simulink model "Dynamic_RR_2019b"  (Simulink 10.0)
settings: Solver=VariableStepAuto  StartTime=0.0  StopTime=1000  FixedStep=1e-2  RelTol=1e-3
undefined symbols (not defined in the file or in its folder): a_11, a_12, b_11, b_12, pi_param, pi_param_hat_0, q0_1, q0_2, qInitial_0, wf
libraries: dspfactors x1
settings Model: Creator=Stefano  LastModifiedBy=dnann
settings DataIOCC: SaveFormat=Dataset  ReturnWorkspaceOutputs=on
settings OptimizationCC: LifeSpan=auto
settings DebuggingCC: UnderspecifiedInitializationDetection=Simplified  MergeDetectMultiDrivingBlocksExec=error  SFUnexpectedBacktrackingDiag=error  SFNoUnconditionalDefaultTransitionDiag=error  SFExecutionAtInitializationDiag=warning  ArithmeticOperatorsInVariantConditions=error
settings HardwareCC: ProdBitPerPointer=64  ProdBitPerSizeT=64  ProdBitPerPtrDiffT=64  ProdLargestAtomicFloat=Float  ProdIntDivRoundTo=Zero  ProdEndianess=LittleEndian  ProdWordSize=64  ProdHWDeviceType=Intel->x86-64 (Windows64)
settings ModelReferenceCC: PropagateSignalLabelsOutOfModel=on
settings SFSimCC: SimUseLocalCustomCode=on  CustomCodeUndefinedFunction=FilterOut
settings RTWCC: RTWUseLocalCustomCode=on
settings CodeAppCC: StateflowObjectComments=off
settings GRTTargetCC: TargetLangStandard=C99 (ISO)  CombineOutputUpdateFcns=on  GRTInterface=off
settings ConfigComp: CovMetricSettings=dwe  CovHtmlReporting=off  CovSaveCumulativeToWorkspaceVar=off  CovSaveSingleToWorkspaceVar=off

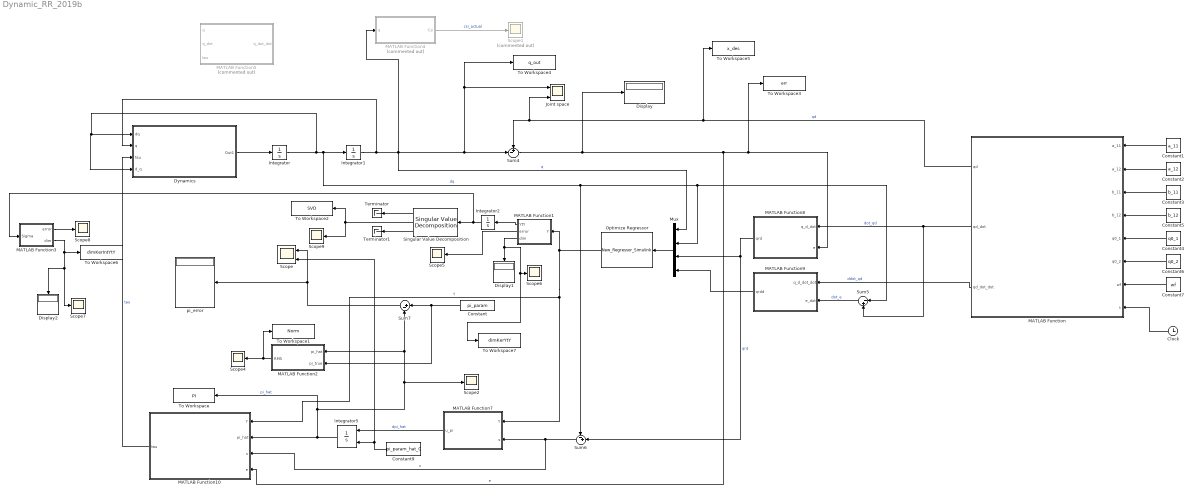
== system Dynamic_RR_2019b ==
  Clock : Clock
  Constant : Constant  Value=pi_param
  Constant1 : Constant  Value=a_11
  Constant2 : Constant  Value=a_12
  Constant3 : Constant  Value=b_11
  Constant4 : Constant  Value=q0_1
  Constant5 : Constant  Value=b_12
  Constant6 : Constant  Value=q0_2
  Constant7 : Constant  Value=wf
  Constant9 : Constant  Value=pi_param_hat_0
  Display : Display
  Display1 : Display
  Display2 : Display
  Dynamics : Subsystem
  Integrator : Integrator  InitialCondition=qInitial_0
  Integrator1 : Integrator  InitialCondition=[0,0]'
  Integrator2 : Integrator
  Integrator5 : Integrator  InitialConditionSource=external
  Joint space : Scope  NumInputPorts=2
  MATLAB Function : MATLAB Function  TreatAsAtomicUnit=on
  MATLAB Function1 : MATLAB Function  TreatAsAtomicUnit=on
  MATLAB Function10 : MATLAB Function  TreatAsAtomicUnit=on
  MATLAB Function2 : MATLAB Function  TreatAsAtomicUnit=on
  MATLAB Function3 : MATLAB Function  TreatAsAtomicUnit=on
  MATLAB Function4 : MATLAB Function  Commented=on  TreatAsAtomicUnit=on
  MATLAB Function5 : MATLAB Function  Commented=on  TreatAsAtomicUnit=on
  MATLAB Function7 : MATLAB Function  TreatAsAtomicUnit=on
  MATLAB Function8 : MATLAB Function  TreatAsAtomicUnit=on
  MATLAB Function9 : MATLAB Function  TreatAsAtomicUnit=on
  Mux : Mux
  "Optimize Regressor " : MATLABFcn  MATLABFcn=New_Regressor_Simulink  OutputDimensions=[2,6]  Output1D=off
  Scope : Scope  NumInputPorts=2
  Scope1 : Scope  Commented=on
  Scope{2,4..9} (7 alike) : Scope
  Singular Value Decomposition : dspfactors/Singular Value Decomposition  wantv=on  wanterr=off  SimulateUsing=Interpreted execution
      settings: SourceProductBaseCode=DS
  Sum4 : Sum  Inputs=+-|
  Sum5 : Sum  Inputs=|-+
  Sum6 : Sum  Inputs=-+|
  Sum7 : Sum  Inputs=|+-
  Terminator : Terminator
  Terminator1 : Terminator
  To Workspace : ToWorkspace  VariableName=PI  SaveFormat=Timeseries  SampleTime=-1
  To Workspace1 : ToWorkspace  VariableName=Norm  SaveFormat=Timeseries  SampleTime=-1
  To Workspace2 : ToWorkspace  VariableName=SVD  SaveFormat=Timeseries  SampleTime=-1
  To Workspace3 : ToWorkspace  VariableName=err  SaveFormat=Timeseries  SampleTime=-1
  To Workspace4 : ToWorkspace  VariableName=q_out  SaveFormat=Timeseries  SampleTime=-1
  To Workspace5 : ToWorkspace  VariableName=x_des  SaveFormat=Timeseries  SampleTime=-1
  To Workspace6 : ToWorkspace  VariableName=dimKerIntYtY  SaveFormat=Timeseries  SampleTime=-1
  To Workspace7 : ToWorkspace  VariableName=dimKerYtY  SaveFormat=Timeseries  SampleTime=-1
  pi_error : Display
  wires:
  Sum6/1 -> MATLAB Function10/3(s), MATLAB Function7/2(s)  "s"
  Sum4/1 -> Display/1, To Workspace3/1, MATLAB Function8/2(e), MATLAB Function10/4(e)  "e"
  Sum5/1 -> MATLAB Function9/2(e_dot)  "dot_e"
  MATLAB Function7/1(u_pi) -> Integrator5/1  "dpi_hat"
  Integrator5/1 -> MATLAB Function10/2(pi_hat), To Workspace/1, Scope2/1, Sum7/2, MATLAB Function2/1(pi_hat)  "pi_hat"
  Integrator/1 -> Sum5/1, Mux/2, Sum6/1, Integrator1/1, Dynamics/1(dq), Dynamics/4(d_q)  "dq"
  Constant9/1 -> Scope/2, Integrator5/2
  MATLAB Function8/1(qrd) -> Sum6/2, Mux/3  "qrd"
  Mux/1 -> "Optimize Regressor "/1
  MATLAB Function9/1(qrdd) -> Mux/4
  Constant/1 -> MATLAB Function2/2(pi_true), Sum7/1
  Sum7/1 -> pi_error/1, Scope/1
  Integrator1/1 -> Dynamics/2(q), Joint space/1, To Workspace4/1, Sum4/2, MATLAB Function4/1(q), Mux/1  "q"
  "Optimize Regressor "/1 -> MATLAB Function10/1(Y), MATLAB Function7/1(Y), MATLAB Function1/1(Y)  "Y"
  MATLAB Function/1(qd) -> To Workspace5/1, Joint space/2, Sum4/1  "qd"
  MATLAB Function/2(qd_dot) -> Sum5/2, MATLAB Function8/1(q_d_dot)  "dot_qd"
  MATLAB Function/3(qd_dot_dot) -> MATLAB Function9/1(q_d_dot_dot)  "ddot_qd"
  MATLAB Function4/1(Csi) -> Scope1/1  "csi_actual"
  Constant1/1 -> MATLAB Function/1(a_11)
  Constant2/1 -> MATLAB Function/2(a_12)
  Constant3/1 -> MATLAB Function/3(b_11)
  Constant5/1 -> MATLAB Function/4(b_12)
  Constant4/1 -> MATLAB Function/5(q0_1)
  Constant6/1 -> MATLAB Function/6(q0_2)
  Constant7/1 -> MATLAB Function/7(wf)
  Clock/1 -> MATLAB Function/8(t)
  MATLAB Function1/1(YtY) -> Integrator2/1
  Singular Value Decomposition/2 -> Scope9/1, To Workspace2/1
  Singular Value Decomposition/1 -> Terminator/1
  Singular Value Decomposition/3 -> Terminator1/1
  Integrator2/1 -> MATLAB Function3/1(Sigma), Singular Value Decomposition/1
  MATLAB Function2/1(RMS) -> To Workspace1/1, Scope4/1
  MATLAB Function10/1(tau) -> Dynamics/3(tau)  "tau"
  Dynamics/1(Out1) -> Integrator/1
  MATLAB Function1/2(error) -> Scope5/1
  MATLAB Function1/3(dim) -> To Workspace7/1, Scope6/1, Display1/1
  MATLAB Function3/2(dim) -> Display2/1, Scope7/1, To Workspace6/1
  MATLAB Function3/1(error) -> Scope8/1

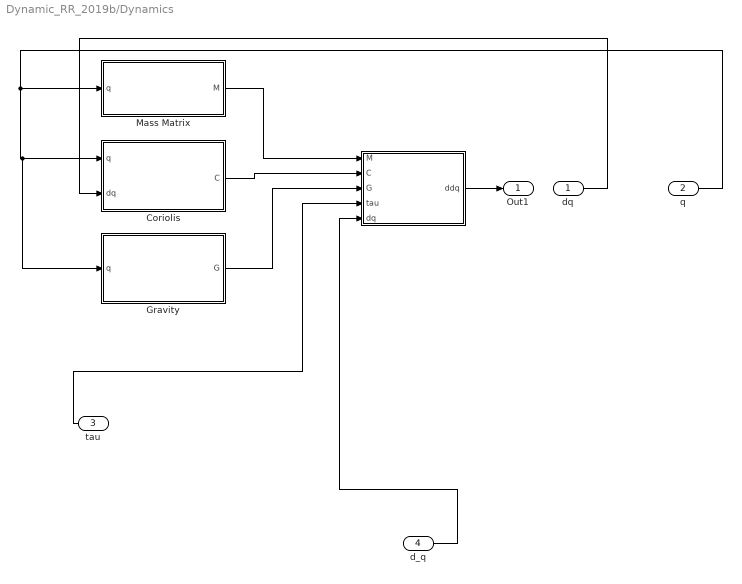
== system Dynamic_RR_2019b/Dynamics ==
  dq : Inport
  q : Inport  Port=2
  tau : Inport  Port=3
  d_q : Inport  Port=4
  " " : MATLAB Function  TreatAsAtomicUnit=on
  "Coriolis " : MATLAB Function  TreatAsAtomicUnit=on
  "Gravity " : MATLAB Function  TreatAsAtomicUnit=on
  "Mass Matrix " : MATLAB Function  TreatAsAtomicUnit=on
  Out1 : Outport
  wires:
  q/1 -> "Gravity "/1(q), "Coriolis "/1(q), "Mass Matrix "/1(q)
  tau/1 -> " "/4(tau)
  "Coriolis "/1(C) -> " "/2(C)
  "Mass Matrix "/1(M) -> " "/1(M)
  "Gravity "/1(G) -> " "/3(G)
  " "/1(ddq) -> Out1/1
  dq/1 -> "Coriolis "/2(dq)
  d_q/1 -> " "/5(dq)

== matlab function MATLAB Function1 ==
  data: Y input double; YtY output double; error output double; dim output double
function [YtY, error,dim] = fcn(Y)

YtY = Y.'*Y;

error = 0;
ker = null(YtY);
dim = 0;

if ker~=0 
    error = 1;
    dim = rank(ker);
end

== matlab function MATLAB Function ==
  data: a_11 input double; qd output double; a_12 input double; b_11 input double; b_12 input double; q0_1 input double; q0_2 input double; wf input double; t input double; qd_dot output double; qd_dot_dot output double
function [qd,qd_dot,qd_dot_dot] = De_Luca_Fourier(a_11,a_12,b_11,b_12,q0_1,q0_2,wf,t)


qd1 = q0_1 - (b_11*cos(t*wf))/wf + (a_11*sin(t*wf))/wf;
qd2 = q0_2 - (b_12*cos(t*wf))/wf + (a_12*sin(t*wf))/wf;

qd = [qd1;qd2];


qd_dot1 = a_11*cos(t*wf) + b_11*sin(t*wf);
qd_dot2 = a_12*cos(t*wf) + b_12*sin(t*wf);

qd_dot = [qd_dot1; qd_dot2];

qd_dot_dot1 = b_11*wf*cos(t*wf) - a_11*wf*sin(t*wf);
qd_dot_dot2 = b_12*wf*cos(t*wf) - a_12*wf*sin(t*wf);

qd_dot_dot = [qd_dot_dot1; qd_dot_dot2];

== matlab function MATLAB Function2 ==
  data: pi_hat input double; RMS output double; pi_true input double
function RMS = Norm(pi_hat,pi_true)

RMS = norm(pi_true - pi_hat);

== matlab function Dynamics/Mass Matrix  ==
  data: q input double; M output double
function M = RR_mass_matrix(q)

% Basic params
g = 9.81;

% Manipulator params
m1 = 1;
m2 = 1;

a1=1;
a2=1;

l1=a1/2;
l2=a2/2;

Izz1 = (1/12)*m1*a1^2;
Izz2 = (1/12)*m2*a2^2;

% Basic expressions for dynamics
Alpha = Izz1 + Izz2 + m1*(l1)^2 + m2*(a1^2+l2^2);
Beta = m2*a1*l2;
Delta = Izz2 +m2*l2^2;

% Mass matrix
M = [Alpha + 2* Beta *cos(q(2)), Delta + Beta *cos(q(2));
     Delta + Beta *cos(q(2)),    Delta];

end

== matlab function MATLAB Function5 ==
  data: q input double; q_dot_dot output double; q_dot input double; tau input double
function q_dot_dot = Forward_Dynamics(q,q_dot,tau)

q1 = q(1);
q2 = q(2);
dq1 = q_dot(1);
dq2 = q_dot(2);
%Properties of the manipulator

m1 = 1;%links mass
m2 = 1;

g = 9.81; %gravity

%COM

l1=0.5;
l2=0.5;

%lenght of the links

a1 = 1;
a2 = 1;

%Inertia respect to the center of mass 

Izz1 = (1/12)*m1*l1^2;
Izz2 = (1/12)*m2*l2^2;

%Inertia Matrix 

b11 = Izz1 + Izz2 + m1*l1^2 + m2*(a1^2 + l2^2 + 2*a1*l2*cos(q2));
b12 = Izz2 + m2*l2*(l2 + a1*cos(q2));
b21 = b12;
b22 = Izz2 + m2*l2^2;


M = [b11, b12; b21, b22];

%Coriolis Matrix

h = -m2*a1*l2*sin(q2);

C = [h*dq2, h*(dq1+dq2);
     -h*dq1,   0];
 
%Gravity matrix

G = [m1*g*l1*cos(q1) + m2*g*(a1*cos(q1) + l2*cos(q1+q2)); m2*g*l2*cos(q1+q2)];

%output

q_dot_dot = inv(M)*([tau(1); tau(2)]- C*[q_dot(1); q_dot(2)] - G);

== matlab function Dynamics/Coriolis  ==
  data: q input double; C output double; dq input double
function C = RR_coriolis_matrix(q, dq)

% Basic params
g = 9.81;

% Manipulator params
m1 = 1;
m2 = 1;

a1=1;
a2=1;

l1=a1/2;
l2=a2/2;

Izz1 = (1/12)*m1*a1^2;
Izz2 = (1/12)*m2*a2^2;

% Basic expressions for dynamics
Alpha = Izz1 + Izz2 + m1*(l1)^2 + m2*(a1^2+l2^2);
Beta = m2*a1*l2;
Delta = Izz2 +m2*l2^2;

% Coriolis matrix
C = [-Beta*sin(q(2))*dq(2), -Beta*sin(q(2))*(dq(1)+dq(2));
     Beta*sin(q(2))*dq(1),   0];

end

== matlab function Dynamics/Gravity  ==
  data: q input double; G output double
function G = RR_gravity_vector(q)

% Basic params
g = 9.81;

% Manipulator params
m1 = 1;
m2 = 1;

a1=1;
a2=1;

l1=a1/2;
l2=a2/2;

Izz1 = (1/12)*m1*a1^2;
Izz2 = (1/12)*m2*a2^2;

% Basic expressions for dynamics
Alpha = Izz1 + Izz2 + m1*(l1)^2 + m2*(a1^2+l2^2);
Beta = m2*a1*l2;
Delta = Izz2 +m2*l2^2;

% Gravity vector
G = [m1*g*l1*cos(q(1)) + m2*g*(a1*cos(q(1)) + l2*cos(q(1)+q(2)));
    m2*g*l2*cos(q(1)+q(2))];

end

== matlab function Dynamics/  ==
  data: M input double; ddq output double; C input double; G input double; tau input double; dq input double
function ddq = Acceleration(M,C,G,tau,dq)

ddq = inv(M)*(tau - C*dq - G);

== matlab function MATLAB Function3 ==
  data: error output double; Sigma input double; dim output double
function [error,dim] = fcn(Sigma)

ker = null(Sigma);
dim = 0;
error=0;

if ker~=0 
    error = 1;
    dim = rank(ker);
end
end

== matlab function MATLAB Function4 ==
  data: q input double; Csi output double
function Csi  = Direct_Kinematics_RR(q)

%INPUT: q(1) = q1;
%       q(2) = q2;

%OUTPUT: px = position along x axis
%        py = position along y axis

%Link's lenght

l1 = 1;
l2 = 1;

px = l1 * cos(q(1)) + l2 * cos(q(1)+q(2));
py = l1 * sin(q(1)) + l2 * sin(q(1)+q(2));

Csi = [px; py];
end

== matlab function MATLAB Function10 ==
  data: Y input double; tau output double; pi_hat input double; s input double; e input double
function tau = Back_Stepping_Control_Law(Y,pi_hat,s,e)

Kd = 12 * eye(2);
Kp = 15 * eye(2);

tau = Y * pi_hat + Kd * s + Kp * e;

end

== matlab function MATLAB Function7 ==
  data: Y input double; u_pi output double; s input double
function u_pi = Update_Law(Y,s)

R = 40 * eye(6,6);
u_pi = inv(R)*(Y')*s;
end

== matlab function MATLAB Function8 ==
  data: q_d_dot input double; qrd output double; e input double
function qrd = q_r_dot(q_d_dot,e)

lambda = 7 * eye(2);
qrd = q_d_dot + lambda * e;

end

== matlab function MATLAB Function9 ==
  data: q_d_dot_dot input double; qrdd output double; e_dot input double
function qrdd = q_r_dot_dot(q_d_dot_dot,e_dot)

lambda = 7 * eye(2);
qrdd = q_d_dot_dot + lambda*e_dot;

end
